simulink model "Movement"  (R2015a)
settings: Solver=ode3  StartTime=0.0  StopTime=10  FixedStep=0.01  RelTol=1e-3
settings Model: Creator=Nick  LastModifiedBy=Nick

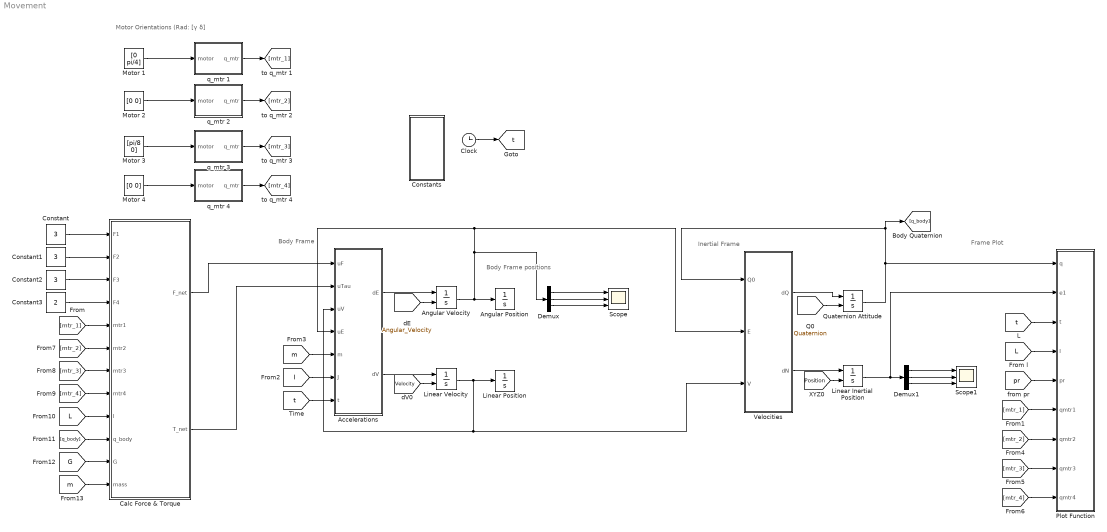
== system Movement ==
  note: Motor Orientations
      | (Rad: [γ δ]
  note: Frame Plot
  note: Inertial Frame
  note: Body Frame
      | positions
  note: Body Frame
  Accelerations : MATLAB Function  TreatAsAtomicUnit=on
  Angular Position : Integrator
  Angular Velocity : Integrator  InitialConditionSource=external
  Calc Force & Torque : MATLAB Function  TreatAsAtomicUnit=on
  Clock : Clock
  Constant : Constant  Value=3
  Constant1 : Constant  Value=3
  Constant2 : Constant  Value=3
  Constant3 : Constant  Value=2
  Constants : Subsystem
  Demux : Demux  Outputs=3
  Demux1 : Demux  Outputs=3
  Linear Inertial Position : Integrator  InitialConditionSource=external
  Linear Position : Integrator
  Linear Velocity : Integrator  InitialConditionSource=external
  Motor 1 : Constant  Value=[0 pi/4]
  Motor 2 : Constant  Value=[0 0]
  Motor 3 : Constant  Value=[pi/8 0]
  Motor 4 : Constant  Value=[0 0]
  Plot Function : MATLAB Function  TreatAsAtomicUnit=on
  Quaternion Attitude : Integrator  InitialConditionSource=external  ContinuousStateAttributes='Quaternion'
  Scope : Scope  NumInputPorts=3
      settings: YMin=-5~-5~-5  YMax=5~5~5
  Scope1 : Scope  NumInputPorts=3
      settings: YMin=-5~-5~-5  YMax=5~5~5
  Velocities : MATLAB Function  TreatAsAtomicUnit=on
  q_mtr 1 : MATLAB Function  TreatAsAtomicUnit=on
  q_mtr 2 : MATLAB Function  TreatAsAtomicUnit=on
  q_mtr 3 : MATLAB Function  TreatAsAtomicUnit=on
  q_mtr 4 : MATLAB Function  TreatAsAtomicUnit=on
  tag scope: t=global
  wires:
  [L] -> Plot Function/4(l)
  [pr] -> Plot Function/5(pr)
  Clock/1 -> [t]
  [t] -> Plot Function/3(t)
  [t] -> Accelerations/7(t)
  [I] -> Accelerations/6(J)
  [m] -> Accelerations/5(m)
  Accelerations/1(dE) -> Angular Velocity/1
  Angular Velocity/1 -> Demux/1, Accelerations/4(uE), Velocities/2(E), Angular Position/1
  Accelerations/2(dV) -> Linear Velocity/1
  Linear Velocity/1 -> Accelerations/3(uV), Velocities/3(V), Linear Position/1
  Demux/1 -> Scope/1
  Demux/2 -> Scope/2
  Demux/3 -> Scope/3
  Demux1/1 -> Scope1/1
  Demux1/2 -> Scope1/2
  Demux1/3 -> Scope1/3
  [Velocity] -> Linear Velocity/2
  [Angular_Velocity] -> Angular Velocity/2
  Velocities/2(dN) -> Linear Inertial Position/1
  [Position] -> Linear Inertial Position/2
  Linear Inertial Position/1 -> Demux1/1, Plot Function/2(e1)
  [Quaternion] -> Quaternion Attitude/2
  Velocities/1(dQ) -> Quaternion Attitude/1
  Quaternion Attitude/1 -> [q_body], Velocities/1(Q0), Plot Function/1(q)
  Motor 1/1 -> q_mtr 1/1(motor)
  Motor 2/1 -> q_mtr 2/1(motor)
  Motor 3/1 -> q_mtr 3/1(motor)
  Motor 4/1 -> q_mtr 4/1(motor)
  q_mtr 1/1(q_mtr) -> [mtr_1]
  q_mtr 4/1(q_mtr) -> [mtr_4]
  q_mtr 3/1(q_mtr) -> [mtr_3]
  q_mtr 2/1(q_mtr) -> [mtr_2]
  [mtr_1] -> Plot Function/6(qmtr1)
  [mtr_2] -> Plot Function/7(qmtr2)
  [mtr_3] -> Plot Function/8(qmtr3)
  [mtr_4] -> Plot Function/9(qmtr4)
  [mtr_1] -> Calc Force & Torque/5(mtr1)
  [mtr_2] -> Calc Force & Torque/6(mtr2)
  [mtr_3] -> Calc Force & Torque/7(mtr3)
  [mtr_4] -> Calc Force & Torque/8(mtr4)
  Constant/1 -> Calc Force & Torque/1(F1)
  Constant1/1 -> Calc Force & Torque/2(F2)
  Constant2/1 -> Calc Force & Torque/3(F3)
  Constant3/1 -> Calc Force & Torque/4(F4)
  Calc Force & Torque/1(F_net) -> Accelerations/1(uF)
  Calc Force & Torque/2(T_net) -> Accelerations/2(uTau)
  [L] -> Calc Force & Torque/9(l)
  [q_body] -> Calc Force & Torque/10(q_body)
  [G] -> Calc Force & Torque/11(G)
  [m] -> Calc Force & Torque/12(mass)

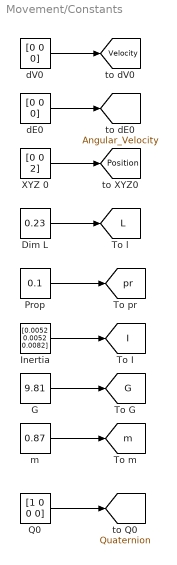
== system Movement/Constants ==
  Dim L : Constant  Value=0.23
  G : Constant  Value=9.81
  Inertia : Constant  Value=[0.0052 0.0052 0.0082]
  Prop : Constant  Value=0.1
  Q0 : Constant  Value=[1 0 0 0]
  XYZ 0 : Constant  Value=[0 0 2]
  dE0 : Constant  Value=[0 0 0]
  dV0 : Constant  Value=[0 0 0]
  m : Constant  Value=0.87
  tag scope: Angular_Velocity=global, G=global, I=global, L=global, Position=global, Quaternion=global, Velocity=global, m=global, pr=global
  wires:
  XYZ 0/1 -> [Position]
  Dim L/1 -> [L]
  Prop/1 -> [pr]
  Inertia/1 -> [I]
  G/1 -> [G]
  m/1 -> [m]
  dV0/1 -> [Velocity]
  dE0/1 -> [Angular_Velocity]
  Q0/1 -> [Quaternion]

== matlab function Movement/Calc Force & Torque ==
  data: F_net output; F1 input; F2 input; F3 input; F4 input; mtr1 input; mtr2 input; mtr3 input; mtr4 input; T_net output; l input; q_body input; G input; mass input
function [F_net,T_net] = motor_dynamics(F1,F2,F3,F4,mtr1,mtr2,mtr3,mtr4,l,q_body,G,mass)
%%Gravity Vector -> Inertial Frame
F_g_w = [0 0 0 -mass*G];
%%Body Frame Quaternion
Q_b = quatnormalize([q_body(1) q_body(2) q_body(3) q_body(4)]);
Q_b_conj = quatconj(Q_b);
%%Motor Forces -> Motor Frames (respectively)
q_F1 = [0 0 0 F1];
q_F2 = [0 0 0 F2];
q_F3 = [0 0 0 F3];
q_F4 = [0 0 0 F4];
%%Motor Frame quaternions
qmtr1 = quatnormalize([mtr1(1) mtr1(2) mtr1(3) mtr1(4)]);
qmtr1_conj = quatconj(qmtr1);
qmtr2 = quatnormalize([mtr2(1) mtr2(2) mtr2(3) mtr2(4)]);
qmtr2_conj = quatconj(qmtr2);
qmtr3 = quatnormalize([mtr3(1) mtr3(2) mtr3(3) mtr3(4)]);
qmtr3_conj = quatconj(qmtr3);
qmtr4 = quatnormalize([mtr4(1) mtr4(2) mtr4(3) mtr4(4)]);
qmtr4_conj = quatconj(qmtr4);
%%Motor Forces -> Body Frame
q_F1_b = quatmultiply((quatmultiply(qmtr1_conj,q_F1)),qmtr1);
q_F2_b = quatmultiply((quatmultiply(qmtr2_conj,q_F2)),qmtr2);
q_F3_b = quatmultiply((quatmultiply(qmtr3_conj,q_F3)),qmtr3);
q_F4_b = quatmultiply((quatmultiply(qmtr4_conj,q_F4)),qmtr4);
q_F_m = q_F1_b + q_F2_b + q_F3_b + q_F4_b; 
%%Gravity Vector -> Body Frame
F_g_b = quatmultiply((quatmultiply(Q_b,F_g_w)),Q_b_conj);
%%F_net summed together 
q_F = q_F_m + F_g_b; % + D
F_net = [q_F(2) q_F(3) q_F(4)];
%%Differential Torques -> Body Frame
T_diff_x = l*q_F1_b(4) - l*q_F3_b(4);
T_diff_y = l*q_F2_b(4) - l*q_F4_b(4);
T_diff_z = l*q_F1_b(2) - l*q_F3_b(2) + l*q_F2_b(1) - l*q_F4_b(1);
T_diff = [T_diff_x T_diff_y T_diff_z];
%%T_net Summed together
T = T_diff; % + G + M
disp(T);
T_net = [T(1) T(2) T(3)];
end

== matlab function Movement/Accelerations ==
  data: uF input; uTau input; uV input; uE input; m input; J input; t input; dE output; dV output
function [dE,dV]= Dynamics(uF,uTau,uV,uE,m,J,t) %#ok<*INUSD>
mass = m; %variable mass
%%Mass Moment of Inertia
J_x = J(1);
J_y = J(2);
J_z = J(3); %Kg.Nm
%%control action
%%All in F_b
%%Force Inputs
f_x = uF(1);
f_y = uF(2);
f_z = uF(3);
F = [f_x f_y f_z]; %N
%%Torque Inputs
t_phi = uTau(1);
t_theta = uTau(2);
t_rho = uTau(3);
Tau = [t_phi t_theta t_rho]; %Nm
disp(uTau);
%%current state translational velocity
u = uV(1);
v = uV(2);
w = uV(3);
V = [u v w]; %m.s^-1
%%current state angular velocity
p = uE(1);
q = uE(2);
r = uE(3);
E = [p q r]; %rad.s^-1
%%Angular accelerations in Body Frame
dp = (1/J_x)*((J_y-J_z)*q*r+t_phi);
dq = (1/J_y)*((J_z-J_x)*p*r+t_theta);
dr = (1/J_z)*((J_x-J_y)*p*q+t_rho);
dE = zeros(3,1); %rad.s^-2
dE(1)=dp;
dE(2)=dq;
dE(3)=dr;
%%Linear accelerations in Body Frame
dV = cross(E,V)+(1/mass)*F; %m.s^-2
%Integrals take place outside dynamics function
end

== matlab function Movement/Plot Function ==
  data: q input; e1 input; t input; l input; pr input; qmtr1 input; qmtr2 input; qmtr3 input; qmtr4 input
function plot(q,e1,t,l,pr,qmtr1,qmtr2,qmtr3,qmtr4)
%Input t
%CG Cartesian Co-ordinates
X = e1(1); %X Position
Y = e1(2); %Y Position
Z = e1(3); %Z Position
%Calculate Motor Positions relative to 0;0;0
%l may be variable
XYmtr1 = ([l 0 0]);
XYmtr2 = ([0 l 0]);
XYmtr3 = ([-l 0 0]);
XYmtr4 = ([0 -l 0]);
%%Calculate Body Attidue (Normal Vector)
Q = quatnormalize(q.'); %Body Quaternion, read from d/dt(Q)
Q_conj = quatconj(Q);   %Quaternion conjugate
N_b = [0 0 1];      %normal vector in Body frame
L_b = [0 N_b(1) N_b(2) N_b(3)]; %Build normal quaternion
L1 = quatmultiply(Q_conj,L_b);
L2 = quatmultiply(L1,Q);    %Normal rotated by Body Quaternion
N_w = [L2(2) L2(3) L2(4)];  %Normal vector in inertial frame
%%Calculate Motor 1 Attitudes
Q_XYmtr1 = [0 XYmtr1(1) XYmtr1(2) XYmtr1(3)]; %XYZ position of motor 1 from CG
L1 = quatmultiply(Q_conj,Q_XYmtr1);
L2 = quatmultiply(L1,Q);    %Rotate rotor arm by body quaternion
mtr1_w = e1.' + [L2(2) L2(3) L2(4)]; %Calculate new XYZ position using attitude quaternion
L_1 = [0 0 0 1];       %k considered to be normal for motor 1 (Force acting just in the Z-direction)
Q_mtr1 = [qmtr1(1) qmtr1(2) qmtr1(3) qmtr1(4)]; %Calculate motor 1 attitude from motor 1 quaternion
Q_mtr1_conj = quatconj(Q_mtr1);
L1 = quatmultiply(Q_mtr1_conj,L_1);
L2 = quatmultiply(L1,Q_mtr1);
L3 = quatmultiply(Q_conj,L2);
L4 = quatmultiply(L3,Q);
mtr1_N = [L4(2) L4(3) L4(4)]; %Motor 1 Normal Vector
%%Calculate Motor 3 Attitudes
Q_XYmtr3 = [0 XYmtr3(1) XYmtr3(2) XYmtr3(3)];
L1 = quatmultiply(Q_conj,Q_XYmtr3);
L2 = quatmultiply(L1,Q);
mtr3_w = e1.' + [L2(2) L2(3) L2(4)];
L_3 = [0 0 0 1];
Q_mtr3 = [qmtr3(1) qmtr3(2) qmtr3(3) qmtr3(4)]; %Calculate motor 3 attitude from motor 3 quaternion
Q_mtr3_conj = quatconj(Q_mtr3);
L1 = quatmultiply(Q_mtr3_conj,L_3);
L2 = quatmultiply(L1,Q_mtr3);
L3 = quatmultiply(Q_conj,L2);
L4 = quatmultiply(L3,Q);
mtr3_N = [L4(2) L4(3) L4(4)]; %Motor 3 Normal Vector
%%Calculate Motor 2 Attitudes
Q_XYmtr2 = [0 XYmtr2(1) XYmtr2(2) XYmtr2(3)];
L1 = quatmultiply(Q_conj,Q_XYmtr2);
L2 = quatmultiply(L1,Q);
mtr2_w = e1.' + [L2(2) L2(3) L2(4)];
L_2 = [0 0 0 1];
Q_mtr2 = [qmtr2(1) qmtr2(2) qmtr2(3) qmtr2(4)]; %Calculate motor 2 attitude from motor 2 quaternion
Q_mtr2_conj = quatconj(Q_mtr2);
L1 = quatmultiply(Q_mtr2_conj,L_2);
L2 = quatmultiply(L1,Q_mtr2);
L3 = quatmultiply(Q_conj,L2);
L4 = quatmultiply(L3,Q);
mtr2_N = [L4(2) L4(3) L4(4)]; %Motor 2 Normal Vector
%%Calculate Motor 4 Attitudes
Q_XYmtr4 = [0 XYmtr4(1) XYmtr4(2) XYmtr4(3)];
L1 = quatmultiply(Q_conj,Q_XYmtr4);
L2 = quatmultiply(L1,Q);
mtr4_w = e1.' + [L2(2) L2(3) L2(4)];
L_4 = [0 0 0 1];
Q_mtr4 = [qmtr4(1) qmtr4(2) qmtr4(3) qmtr4(4)]; %Calculate motor 2 attitude from motor 2 quaternion
Q_mtr4_conj = quatconj(Q_mtr4);
L1 = quatmultiply(Q_mtr4_conj,L_4);
L2 = quatmultiply(L1,Q_mtr4);
L3 = quatmultiply(Q_conj,L2);
L4 = quatmultiply(L3,Q);
mtr4_N = [L4(2) L4(3) L4(4)]; %Motor 2 Normal Vector
%%Open Figure if first time instance
if(t==0);
    fig = figure();
    hold on;
    grid on;
end
%%Clear and Construct Figure
hold off;
clf();
xlim([-1 5]);
ylim([-1 5]);
zlim([0 5]);
view([4 4 5]);
grid on;
hold on;
%%Display Time
%disp(t);
%%Plot Quad Function
plotCircle3D([X Y 0],[0 0 1],(l),'black');
plot3(([mtr1_w(1) mtr3_w(1)]),([mtr1_w(2) mtr3_w(2)]),([mtr1_w(3) mtr3_w(3)]),'LineWidth',1,'Color','Blue');
plot3(([mtr2_w(1) mtr4_w(1)]),([mtr2_w(2) mtr4_w(2)]),([mtr2_w(3) mtr4_w(3)]),'LineWidth',1,'Color','Blue');
plotCircle3D(mtr1_w,mtr1_N,pr,'red');
plotCircle3D(mtr2_w,mtr2_N,pr,'red');
plotCircle3D(mtr3_w,mtr3_N,pr,'red');
plotCircle3D(mtr4_w,mtr4_N,pr,'red');
plotCircle3D([X Y Z],N_w,(l+pr),'green');
%%
end

== matlab function Movement/Velocities ==
  data: Q0 input; dQ output; E input; V input; dN output
function [dQ,dN] = inertialdynamics(Q0,E,V)
%#codegen
V1 = V.';
qE = [0 E(1) E(2) E(3)];
Q = quatnormalize(Q0.');
Q_conj = quatconj(Q);
dQ=(1/2)*quatmultiply(Q,qE);
%ndQ = quatnormalize(dQ);
V2 = [0 V1(1) V1(2) V1(3)];
L1 = quatmultiply(Q_conj,V2);
L2 = quatmultiply(L1,Q);
dN = [L2(2) L2(3) L2(4)];
end

== matlab function Movement/q_mtr 1 ==
  data: motor input; q_mtr output
function q_mtr = quat_convert(motor)
q_mtr = zeros(1,4);
gamma = motor(1);
delta = motor(2);
q_gamma = [cos(gamma/2) 0 sin(gamma/2) 0];
q_delta = [cos(delta/2) sin(delta/2) 0 0];
q = quatmultiply(q_gamma,q_delta);
q_mtr = quatnormalize(q);
end

== matlab function Movement/q_mtr 2 ==
  data: motor input; q_mtr output
function q_mtr = quat_convert(motor)
q_mtr = zeros(1,4);
gamma = motor(1);
delta = motor(2);
q_gamma = [cos(gamma/2) 0 sin(gamma/2) 0];
q_delta = [cos(delta/2) sin(delta/2) 0 0];
q = quatmultiply(q_gamma,q_delta);
q_mtr = quatnormalize(q);
end

== matlab function Movement/q_mtr 3 ==
  data: motor input; q_mtr output
function q_mtr = quat_convert(motor)
q_mtr = zeros(1,4);
gamma = motor(1);
delta = motor(2);
q_gamma = [cos(gamma/2) 0 sin(gamma/2) 0];
q_delta = [cos(delta/2) sin(delta/2) 0 0];
q = quatmultiply(q_gamma,q_delta);
q_mtr = quatnormalize(q);
end

== matlab function Movement/q_mtr 4 ==
  data: motor input; q_mtr output
function q_mtr = quat_convert(motor)
q_mtr = zeros(1,4);
gamma = motor(1);
delta = motor(2);
q_gamma = [cos(gamma/2) 0 sin(gamma/2) 0];
q_delta = [cos(delta/2) sin(delta/2) 0 0];
q = quatmultiply(q_gamma,q_delta);
q_mtr = quatnormalize(q);
end
